simulink model "controller_archive"  (R2022b)
settings: Solver=ode4  StartTime=0.0  StopTime=4  FixedStep=0.001  RelTol=1e-3
PreLoadFcn:
  | global m1 m2 l g m1_hat m2_hat;
  | m1 = 2;
  | m2 = 2;
  | m1_hat = 0.97*m1;
  | m2_hat = 0.97*m2;
  | l = 1;
  | g = 9.81;
  | 
  | kd = 200;
  | md = m1_hat;
  | dd = 2*0.7*sqrt(kd*md);
  | 
  | Kd = [kd,0;0,kd];
  | Md = [md,0;0,md];
  | Dd = [dd,0;0,dd];
  | 
  | p = 10^6;
  | d = 2*0.7*sqrt(p);
  | 
  | P = [p,0;0,p];
  | D = [d,0;0,d];
  | 
  | D_hold = D;
  | P_hold = P;
  | 
  | ke = 300;
  | Ke = [ke,0;0,0];
  | 
  | Fc = 1;
  | cv = 4;
  | 
  | delta = 0.01;
  | 
  | x0 = [0.95,0.95];
  | dx0 = [0;0];
  | 
  | n_pow = 0.001;
  | 
  | wall = 0.8;
  | 
  | delay = 2;
libraries: simulink x1, bbblueBasicLib x1
settings Model: SimulationMode=external  ExtModeTrigDuration=100  Creator=Nick  LastModifiedBy=Nick
settings SolverCC: PositivePriorityOrder=on  AutoInsertRateTranBlk=on  InsertRTBMode=Always
settings OptimizationCC: EnhancedBackFolding=on  PassReuseOutputArgsAs=Individual arguments  ZeroExternalMemoryAtStartup=off  ZeroInternalMemoryAtStartup=off  MaxStackSize=64  OptimizeBlockOrder=speed  DifferentSizesBufferReuse=on  OptimizationCustomize=off  EfficientTunableParamExpr=on
settings DebuggingCC: ParameterTunabilityLossMsg=error  UnconnectedInputMsg=warning  UnconnectedOutputMsg=warning  UnconnectedLineMsg=warning
settings HardwareCC: ProdBitPerPointer=32  ProdBitPerSizeT=32  ProdBitPerPtrDiffT=32  ProdLargestAtomicInteger=Long  ProdLargestAtomicFloat=Double  ProdWordSize=32  ProdHWDeviceType=ARM Compatible->ARM Cortex  UseEmbeddedCoderFeatures=off
settings ModelReferenceCC: EnableRefExpFcnMdlSchedulingChecks=on
settings SFSimCC: SimUserIncludeDirs=C:\Users\Nick\Documents\Github\beaglebone-epos-can\simulink\placeholders  MATLABDynamicMemAlloc=off
settings SFSimCC: SimCustomHeaderCode=|
  | #include "init_can.h"
  | #include "get_encoder.h"
  | #include "set_motor.h"
  | #include "print_input.h"
  | #include "stop_motor.h"
settings SFSimCC: SimUserSources=|
  | C:\Users\Nick\Documents\Github\beaglebone-epos-can\simulink\placeholders\init_can.c
  | C:\Users\Nick\Documents\Github\beaglebone-epos-can\simulink\placeholders\set_motor.c
  | C:\Users\Nick\Documents\Github\beaglebone-epos-can\simulink\placeholders\get_encoder.c
  | C:\Users\Nick\Documents\Github\beaglebone-epos-can\simulink\placeholders\print_input.c
  | C:\Users\Nick\Documents\Github\beaglebone-epos-can\simulink\placeholders\stop_motor.c
settings RTWCC: Description=Embedded Coder  SystemTargetFile=ert.tlc  HardwareBoard=BeagleBone Blue  TLCOptions="-aInlineSetEventsForThisBaseRateFcn=TLC_FALSE -aSuppressMultiTaskScheduler=TLC_FALSE  -aRateBasedStepFcn=0"  TemplateMakefile=ert_default_tmf  RTWUseSimCustomCode=on  CustomInclude=C:\Users\Nick\Documents\Github\beaglebone-epos-can\simulink\placeholders  Toolchain=GNU GCC BeagleBone Blue  BuildConfiguration=Faster Runs  DLArmComputeVersion=19.05
settings RTWCC: CustomHeaderCode=|
  | #include "init_can.h"
  | #include "get_encoder.h"
  | #include "set_motor.h"
  | #include "print_input.h"
  | #include "stop_motor.h"
settings RTWCC: CustomSource=|
  | C:\Users\Nick\Documents\Github\beaglebone-epos-can\simulink\placeholders\init_can.c
  | C:\Users\Nick\Documents\Github\beaglebone-epos-can\simulink\placeholders\set_motor.c
  | C:\Users\Nick\Documents\Github\beaglebone-epos-can\simulink\placeholders\get_encoder.c
  | C:\Users\Nick\Documents\Github\beaglebone-epos-can\simulink\placeholders\print_input.c
  | C:\Users\Nick\Documents\Github\beaglebone-epos-can\simulink\placeholders\stop_motor.c
settings CodeAppCC: ForceParamTrailComments=on  IgnoreCustomStorageClasses=off  OperatorAnnotations=on  SimulinkDataObjDesc=on  SFDataObjDesc=on  InsertBlockDesc=on
settings ERTTargetCC: SupportNonInlinedSFcns=on  SupportVariableSizeSignals=on

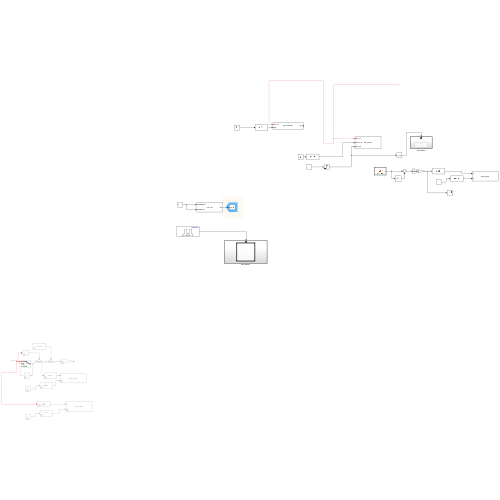
[thumbnail: Simulink's stored preview of the top-level diagram]
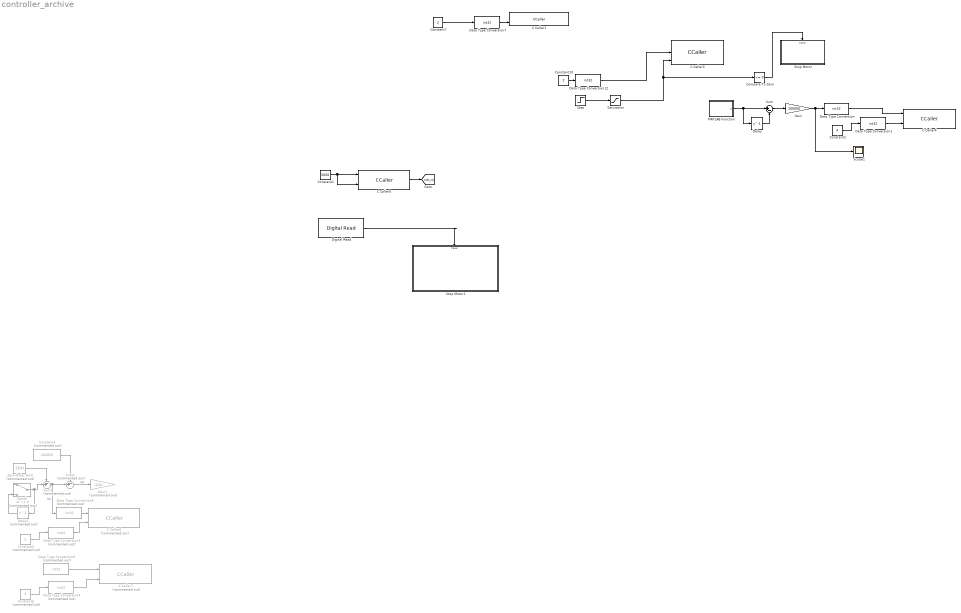
== system controller_archive ==
  C Caller1 : CCaller  FunctionName=get_encoder  PortSpecificationStruct="%)30     .    : 4   8    (     @         %    \"     ,    !     0         %  0 \"0    $    _    07)G3F%M90  4&]R=$YA;64 4V-O<&4     26YD97@     5'EP90      4VEZ90      27-';&]B86P   X    X    !@    @    $          4    (     0    8    !         !     &    <&1O7VED   .    .     8    (    !          %    \"     $    &     0         0    !@   '!D;U]I9   #@   #@    &    \"     0         !0    @    !    !0    $         $     4   !);G!U=     X    X    !@    @    &          4    (     0    $    !          D    (               .    .     8    (    !          %    \"     $    %     0         0    !0   &EN=#,R    #@   #     &    \"     0         !0    @    !     0    $         $  ! #$    .    ,     8    (    \"0(        %    \"     $    !     0         \"  $       X    P    !@    @    $          4    (     0    0    !         !  ! !S:7IE#@   #     &    \"     0         !0    @    !    !     $         $  $ '-I>F4.    .     8    (    !          %    \"     $    %     0         0    !0   $EN<'5T    #@   #@    &    \"     8         !0    @    !     0    $         \"0    @           #P/PX    X    !@    @    $          4    (     0    4    !         !     %    :6YT,S(    .    ,     8    (    !          %    \"     $    !     0         0  $ ,0    X    P    !@    @    ) @        4    (     0    $    !          (  0      #@   #     &    \"     0         !0    @    !     P    $         $  # '!O<P .    ,     8    (    !          %    \"     $    #     0         0  , <&]S  X    X    !@    @    $          4    (     0    8    !         !     &    3W5T<'5T   .    .     8    (    !@         %    \"     $    !     0         )    \"               #@   #@    &    \"     0         !0    @    !    !@    $         $     8   !D;W5B;&4   X    P    !@    @    $          4    (     0    $    !         !   0 R    #@   #     &    \"     D\"        !0    @    !     0    $          @ !"  SampleTime=0.01
  C Caller3 : CCaller  FunctionName=set_motor  PortSpecificationStruct="%)30     .    B 4   8    (     @         %    \"     ,    !     0         %  0 \"0    $    _    07)G3F%M90  4&]R=$YA;64 4V-O<&4     26YD97@     5'EP90      4VEZ90      27-';&]B86P   X    X    !@    @    $          4    (     0    8    !         !     &    <&1O7VED   .    .     8    (    !          %    \"     $    &     0         0    !@   '!D;U]I9   #@   #@    &    \"     0         !0    @    !    !0    $         $     4   !);G!U=     X    X    !@    @    &          4    (     0    $    !          D    (               .    .     8    (    !          %    \"     $    %     0         0    !0   &EN=#,R    #@   #     &    \"     0         !0    @    !     0    $         $  ! #$    .    ,     8    (    \"0(        %    \"     $    !     0         \"  $       X    X    !@    @    $          4    (     0    @    !         !     (    ;6]T;W)?:60.    .     8    (    !          %    \"     $    (     0         0    \"    &UO=&]R7VED#@   #@    &    \"     0         !0    @    !    !0    $         $     4   !);G!U=     X    X    !@    @    &          4    (     0    $    !          D    (            \\#\\.    .     8    (    !          %    \"     $    %     0         0    !0   &EN=#,R    #@   #     &    \"     0         !0    @    !     0    $         $  ! #$    .    ,     8    (    \"0(        %    \"     $    !     0         \"  $       X    X    !@    @    $          4    (     0    <    !         !     '    <V5T7W9A;  .    .     8    (    !          %    \"     $    '     0         0    !P   '-E=%]V86P #@   #@    &    \"     0         !0    @    !    !0    $         $     4   !);G!U=     X    X    !@    @    &          4    (     0    $    !          D    (             $ .    .     8    (    !          %    \"     $    &     0         0    !@   &1O=6)L90  #@   #     &    \"     0         !0    @    !     0    $         $  ! #$    .    ,     8    (    \"0(        %    \"     $    !     0         \"  $"  SampleTime=0.01
  C Caller4 : CCaller  FunctionName=print_input  PortSpecificationStruct="%)30     .    N ,   8    (     @         %    \"     (    !     0         %  0 \"0    $    _    07)G3F%M90  4&]R=$YA;64 4V-O<&4     26YD97@     5'EP90      4VEZ90      27-';&]B86P   X    P    !@    @    $          4    (     0    $    !         !   0!A    #@   #     &    \"     0         !0    @    !     0    $         $  ! &$    .    .     8    (    !          %    \"     $    %     0         0    !0   $EN<'5T    #@   #@    &    \"     8         !0    @    !     0    $         \"0    @               X    X    !@    @    $          4    (     0    4    !         !     %    :6YT,S(    .    ,     8    (    !          %    \"     $    !     0         0  $ ,0    X    P    !@    @    ) @        4    (     0    $    !          (  0      #@   #     &    \"     0         !0    @    !     @    $         $  \" &ED   .    ,     8    (    !          %    \"     $    \"     0         0  ( :60   X    X    !@    @    $          4    (     0    4    !         !     %    26YP=70    .    .     8    (    !@         %    \"     $    !     0         )    \"            / _#@   #@    &    \"     0         !0    @    !    !0    $         $     4   !I;G0S,@    X    P    !@    @    $          4    (     0    $    !         !   0 Q    #@   #     &    \"     D\"        !0    @    !     0    $          @ !"  SampleTime=0.001
  C Caller5 : CCaller  FunctionName=init_can  PortSpecificationStruct="%)30     .    > 4   8    (     @         %    \"     ,    !     0         %  0 \"0    $    _    07)G3F%M90  4&]R=$YA;64 4V-O<&4     26YD97@     5'EP90      4VEZ90      27-';&]B86P   X    P    !@    @    $          4    (     0    ,    !         !   P!O=70 #@   #     &    \"     0         !0    @    !     P    $         $  # &]U=  .    .     8    (    !          %    \"     $    &     0         0    !@   $]U='!U=   #@   #@    &    \"     8         !0    @    !     0    $         \"0    @               X    X    !@    @    $          4    (     0    4    !         !     %    :6YT,S(    .    ,     8    (    !          %    \"     $    !     0         0  $ ,0    X    P    !@    @    ) @        4    (     0    $    !          (  0      #@   #@    &    \"     0         !0    @    !    \"     $         $     @   !M87A3<&5E9 X    X    !@    @    $          4    (     0    @    !         !     (    ;6%X4W!E960.    .     8    (    !          %    \"     $    %     0         0    !0   $EN<'5T    #@   #@    &    \"     8         !0    @    !     0    $         \"0    @               X    X    !@    @    $          4    (     0    8    !         !     &    9&]U8FQE   .    ,     8    (    !          %    \"     $    !     0         0  $ ,0    X    P    !@    @    ) @        4    (     0    $    !          (  0      #@   #@    &    \"     0         !0    @    !    \"     $         $     @   !M87A!8V-E; X    X    !@    @    $          4    (     0    @    !         !     (    ;6%X06-C96P.    .     8    (    !          %    \"     $    %     0         0    !0   $EN<'5T    #@   #@    &    \"     8         !0    @    !     0    $         \"0    @           #P/PX    X    !@    @    $          4    (     0    8    !         !     &    9&]U8FQE   .    ,     8    (    !          %    \"     $    !     0         0  $ ,0    X    P    !@    @    ) @        4    (     0    $    !          (  0"  SampleTime=10000
  C Caller6 : CCaller  Commented=on  FunctionName=print_input  PortSpecificationStruct="%)30     .    N ,   8    (     @         %    \"     (    !     0         %  0 \"0    $    _    07)G3F%M90  4&]R=$YA;64 4V-O<&4     26YD97@     5'EP90      4VEZ90      27-';&]B86P   X    P    !@    @    $          4    (     0    $    !         !   0!A    #@   #     &    \"     0         !0    @    !     0    $         $  ! &$    .    .     8    (    !          %    \"     $    %     0         0    !0   $EN<'5T    #@   #@    &    \"     8         !0    @    !     0    $         \"0    @               X    X    !@    @    $          4    (     0    4    !         !     %    :6YT,S(    .    ,     8    (    !          %    \"     $    !     0         0  $ ,0    X    P    !@    @    ) @        4    (     0    $    !          (  0      #@   #     &    \"     0         !0    @    !     @    $         $  \" &ED   .    ,     8    (    !          %    \"     $    \"     0         0  ( :60   X    X    !@    @    $          4    (     0    4    !         !     %    26YP=70    .    .     8    (    !@         %    \"     $    !     0         )    \"            / _#@   #@    &    \"     0         !0    @    !    !0    $         $     4   !I;G0S,@    X    P    !@    @    $          4    (     0    $    !         !   0 Q    #@   #     &    \"     D\"        !0    @    !     0    $          @ !"  SampleTime=0.01
  C Caller7 : CCaller  Commented=on  FunctionName=print_input  PortSpecificationStruct="%)30     .    N ,   8    (     @         %    \"     (    !     0         %  0 \"0    $    _    07)G3F%M90  4&]R=$YA;64 4V-O<&4     26YD97@     5'EP90      4VEZ90      27-';&]B86P   X    P    !@    @    $          4    (     0    $    !         !   0!A    #@   #     &    \"     0         !0    @    !     0    $         $  ! &$    .    .     8    (    !          %    \"     $    %     0         0    !0   $EN<'5T    #@   #@    &    \"     8         !0    @    !     0    $         \"0    @               X    X    !@    @    $          4    (     0    4    !         !     %    :6YT,S(    .    ,     8    (    !          %    \"     $    !     0         0  $ ,0    X    P    !@    @    ) @        4    (     0    $    !          (  0      #@   #     &    \"     0         !0    @    !     @    $         $  \" &ED   .    ,     8    (    !          %    \"     $    \"     0         0  ( :60   X    X    !@    @    $          4    (     0    4    !         !     %    26YP=70    .    .     8    (    !@         %    \"     $    !     0         )    \"            / _#@   #@    &    \"     0         !0    @    !    !0    $         $     4   !I;G0S,@    X    P    !@    @    $          4    (     0    $    !         !   0 Q    #@   #     &    \"     D\"        !0    @    !     0    $          @ !"  SampleTime=0.01
  Compare To Zero : simulink/Logic and Bit Operations/Compare To Zero  relop=<=  OutDataTypeStr=boolean
  Constant1 : Constant  Value=5000
  Constant10 : Constant  Value=2
  Constant2 : Constant  Value=4
  Constant3 : Constant  Commented=on  Value=200000
  Constant4 : Constant  Commented=on  Value=2
  Constant5 : Constant  Commented=on  Value=3
  Constant7 : Constant  Value=2
  Data Type Conversion{,1,7,12} (4 alike) : DataTypeConversion  OutDataTypeStr=int32  SaturateOnIntegerOverflow=off  RndMeth=Floor
  Data Type Conversion{3..6} (4 alike) : DataTypeConversion  Commented=on  OutDataTypeStr=int32  SaturateOnIntegerOverflow=off  RndMeth=Floor
  Delay : Delay  DelayLength=1  InitialCondition=0
  Delay1 : Delay  Commented=on  DelayLength=1  InitialCondition=0
  Digital Read : bbblueBasicLib/Digital Read  Pin=49  Direction=input  GPIOSelect=GPIO3_17  SampleTime=0.1
  Gain : Gain  Gain=100000
  Gain1 : Gain  Commented=on  Gain=-1/20
  MATLAB Function : MATLAB Function  TreatAsAtomicUnit=on
  Saturation : Saturate  UpperLimit=100  LowerLimit=-100
  Scope1 : Scope
  Step : Step  Time=10  Before=75  After=0  SampleTime=0
  Stop Motor : Subsystem  TreatAsAtomicUnit=on
  Stop Motor1 : Subsystem  TreatAsAtomicUnit=on
  Sum : Sum  Inputs=|+-
  Sum1 : Sum  Commented=on  Inputs=-+|
  Sum2 : Sum  Commented=on  Inputs=-+|
  Switch : Switch  Commented=on  Criteria=u2 ~= 0  SaturateOnIntegerOverflow=off  InputSameDT=off
  Zero-Order Hold : ZeroOrderHold  Commented=on  SampleTime=10000
  wires:
  Delay/1 -> Sum/2
  Sum/1 -> Gain/1
  MATLAB Function/1(y) -> Delay/1, Sum/1
  Data Type Conversion/1 -> C Caller4/1
  Gain/1 -> Scope1/1, Data Type Conversion/1
  Data Type Conversion1/1 -> C Caller4/2
  Constant2/1 -> Data Type Conversion1/1
  ? -> Switch/1, Switch/2, Zero-Order Hold/1, Data Type Conversion6/1
  Zero-Order Hold/1 -> Sum1/1
  Sum1/1 -> Data Type Conversion5/1, Sum2/2  "inc"
  Constant3/1 -> Sum2/1
  Sum2/1 -> Gain1/1  "inc"
  Saturation/1 -> Compare To Zero/1, C Caller3/3
  Switch/1 -> Delay1/1, Sum1/2
  Delay1/1 -> Switch/3
  Data Type Conversion3/1 -> C Caller6/2
  Constant4/1 -> Data Type Conversion3/1
  Constant5/1 -> Data Type Conversion4/1
  Data Type Conversion4/1 -> C Caller7/2
  Data Type Conversion5/1 -> C Caller6/1
  Data Type Conversion6/1 -> C Caller7/1
  ? -> C Caller1/1, C Caller3/1
  Constant7/1 -> Data Type Conversion7/1
  Data Type Conversion7/1 -> C Caller1/2
  Constant10/1 -> Data Type Conversion12/1
  Data Type Conversion12/1 -> C Caller3/2
  Step/1 -> Saturation/1
  Compare To Zero/1 -> Stop Motor/Trigger
  Digital Read/1 -> Stop Motor1/Trigger
  Constant1/1 -> C Caller5/2, C Caller5/1
  C Caller5/1 -> [pdo_id]

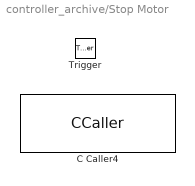
== system controller_archive/Stop Motor ==
  Trigger : TriggerPort  VariantControl=(inherit)
  C Caller4 : CCaller  FunctionName=stop_motor  SampleTime=0.001

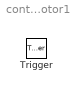
== system controller_archive/Stop Motor1 ==
  Trigger : TriggerPort  VariantControl=(inherit)

== matlab function controller_archive/MATLAB Function ==
  data: y output
function y = sysTime()
    c = datetime('now')
    y=c.Second;
